simulink library "hydro2pumps_lib"  (Simulink 5.0)
settings Model: LastModifiedBy=mato

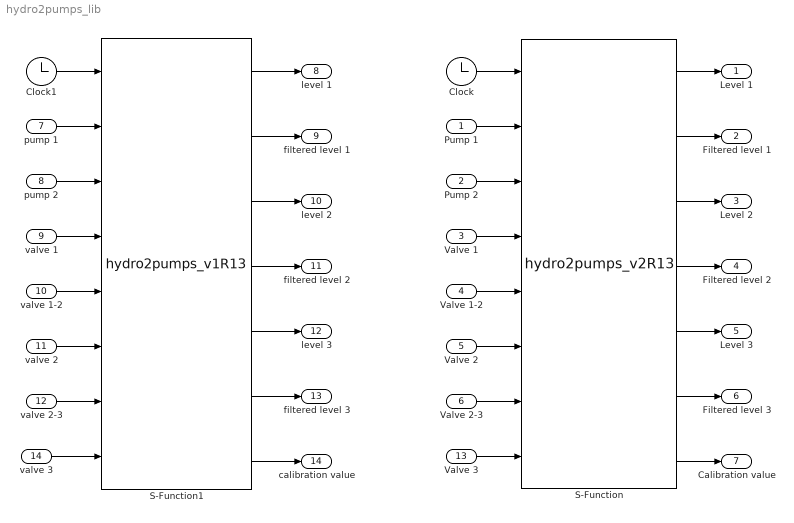
== system hydro2pumps_lib ==
  Pump 1 : Inport
  Pump 2 : Inport  Port=2
  Valve 1 : Inport  Port=3
  Valve 1-2 : Inport  Port=4
  Valve 2 : Inport  Port=5
  Valve 2-3 : Inport  Port=6
  pump 1 : Inport  Port=7
  pump 2 : Inport  Port=8
  valve 1 : Inport  Port=9
  valve 1-2 : Inport  Port=10
  valve 2 : Inport  Port=11
  valve 2-3 : Inport  Port=12
  Valve 3 : Inport  Port=13
  valve 3 : Inport  Port=14
  Clock : Clock
      settings: Decimation=10
  Clock1 : Clock
      settings: Decimation=10
  S-Function : S-Function  Priority=1  FunctionName=hydro2pumps_v2R13  Parameters=com_port, Ts, events_ot, rd_timeout, matlab_prior, warning, printout  mask(hydro2pumps Communication Interface){com_port=COM4, Ts=0.5, events_ot=2, rd_timeout=250, matlab_prior=ABOVE_NORMAL_PRIORITY, warning=on, printout=off}
      mask prompts: com_port "Serial port:"; Ts "Sample time (sec):"; events_ot "Sampling delayed (%):"; rd_timeout "Read timeout (msec, lower than sample time):"; matlab_prior "Matlab priority"; warning "Warning if delayed (error if unchecked)"; printout "Detailed timing and timeout  printout"
      mask help:
      | (c) 2007 Martin Kamensky
      |
      | Serial port - USB serial port number assigned to hydro2pumps system
      |
      | Sampling time (sec) - the lowest working value in Windows is about 0.04 - 0.05 s
      |
      | Sample delayed (%) - number of events (percentually) when simulink loop can take more than time determined by sample time
      |
      | Read timeout (msec) - timeout for reading data from the port (the lowest working value is about 25 ms)
      |
      | Matlab priority :
      | NORMAL_PRIORITY - priority of common Windows application
      | ABOVE_NORMAL_PRIORITY - recommended - higher priority than common Windows application priority
      | HIGH_PRIORITY - recommended - high priority
      | REALTIME_PRIORITY - NOT recommended - takes almost all system resources
      mask init:
      | set_param(bdroot,'FixedStep',get_param(gcb,'Ts'));
      | set_param(bdroot,'Solver','ode1');
      mask StyleString: popup(COM1|COM2|COM3|COM4),edit,edit,edit,popup(NORMAL_PRIORITY|ABOVE_NORMAL_PRIORITY|HIGH_PRIORITY|REALTIME_PRIORITY),checkbox,checkbox
      mask CallbackString:
      | |set_param(bdroot,'FixedStep',get_param(gcb,'Ts'));
      | set_param(bdroot,'Solver','ode1');|||||
  S-Function1 : S-Function  Priority=1  FunctionName=hydro2pumps_v1R13  Parameters=com_port, Ts, events_ot, rd_timeout, matlab_prior, warning, printout  mask(hydro2pumps Communication Interface){com_port=COM4, Ts=0.5, events_ot=2, rd_timeout=250, matlab_prior=ABOVE_NORMAL_PRIORITY, warning=on, printout=off}
      mask prompts: com_port "Serial port:"; Ts "Sample time (sec):"; events_ot "Sampling delayed (%):"; rd_timeout "Read timeout (msec, lower than sample time):"; matlab_prior "Matlab priority"; warning "Warning if delayed (error if unchecked)"; printout "Detailed timing and timeout  printout"
      mask help:
      | (c) 2007 Martin Kamensky
      |
      | Serial port - USB serial port number assigned to hydro2pumps system
      |
      | Sampling time (sec) - the lowest working value in Windows is about 0.04 - 0.05 s
      |
      | Sample delayed (%) - number of events (percentually) when simulink loop can take more than time determined by sample time
      |
      | Read timeout (msec) - timeout for reading data from the port (the lowest working value is about 25 ms)
      |
      | Matlab priority :
      | NORMAL_PRIORITY - priority of common Windows application
      | ABOVE_NORMAL_PRIORITY - recommended - higher priority than common Windows application priority
      | HIGH_PRIORITY - recommended - high priority
      | REALTIME_PRIORITY - NOT recommended - takes almost all system resources
      mask init:
      | set_param(bdroot,'FixedStep',get_param(gcb,'Ts'));
      | set_param(bdroot,'Solver','ode1');
      mask StyleString: popup(COM1|COM2|COM3|COM4),edit,edit,edit,popup(NORMAL_PRIORITY|ABOVE_NORMAL_PRIORITY|HIGH_PRIORITY|REALTIME_PRIORITY),checkbox,checkbox
      mask CallbackString:
      | |set_param(bdroot,'FixedStep',get_param(gcb,'Ts'));
      | set_param(bdroot,'Solver','ode1');|||||
  Level 1 : Outport
  Filtered level 1 : Outport  Port=2
  Level 2 : Outport  Port=3
  Filtered level 2 : Outport  Port=4
  Level 3 : Outport  Port=5
  Filtered level 3 : Outport  Port=6
  Calibration value : Outport  Port=7
  level 1 : Outport  Port=8
  filtered level 1 : Outport  Port=9
  level 2 : Outport  Port=10
  filtered level 2 : Outport  Port=11
  level 3 : Outport  Port=12
  filtered level 3 : Outport  Port=13
  calibration value : Outport  Port=14
  wires:
  S-Function/1 -> Level 1/1
  S-Function/2 -> Filtered level 1/1
  Clock/1 -> S-Function/1
  Pump 1/1 -> S-Function/2
  Pump 2/1 -> S-Function/3
  S-Function/3 -> Level 2/1
  S-Function/4 -> Filtered level 2/1
  S-Function/5 -> Level 3/1
  S-Function/6 -> Filtered level 3/1
  Valve 1/1 -> S-Function/4
  Valve 1-2/1 -> S-Function/5
  Valve 2/1 -> S-Function/6
  Valve 2-3/1 -> S-Function/7
  S-Function/7 -> Calibration value/1
  S-Function1/1 -> level 1/1
  S-Function1/2 -> filtered level 1/1
  Clock1/1 -> S-Function1/1
  pump 1/1 -> S-Function1/2
  pump 2/1 -> S-Function1/3
  S-Function1/3 -> level 2/1
  S-Function1/4 -> filtered level 2/1
  S-Function1/5 -> level 3/1
  S-Function1/6 -> filtered level 3/1
  valve 1/1 -> S-Function1/4
  valve 1-2/1 -> S-Function1/5
  valve 2/1 -> S-Function1/6
  valve 2-3/1 -> S-Function1/7
  S-Function1/7 -> calibration value/1
  Valve 3/1 -> S-Function/8
  valve 3/1 -> S-Function1/8
